simulink model "LQR_2017a"  (R2017a)
settings: Solver=VariableStepAuto  StartTime=0.0  StopTime=4  RelTol=1e-3
values from neighbouring files (symbols this model uses):
  A_obs = A-L*C    [ventilador.m]
  B_obs = [B L]    [ventilador.m]
  C_obs = eye(3)    [ventilador.m]
  D_obs = zeros(3,2)    [ventilador.m]
  K = (tf - t0) / dt    (= 1000)    [pruebaPendulo.m]    (also in ventilador.m = place(A, B, polo_fav))
  Nbar = rscale(sis,K)    [ventilador.m]
undefined symbols (not defined in the file or in its folder): A, B, C, D
settings Model: Creator=jacqu  LastModifiedBy=Gaby
settings SFSimCC: SimUseLocalCustomCode=on
settings RTWCC: RTWUseLocalCustomCode=on

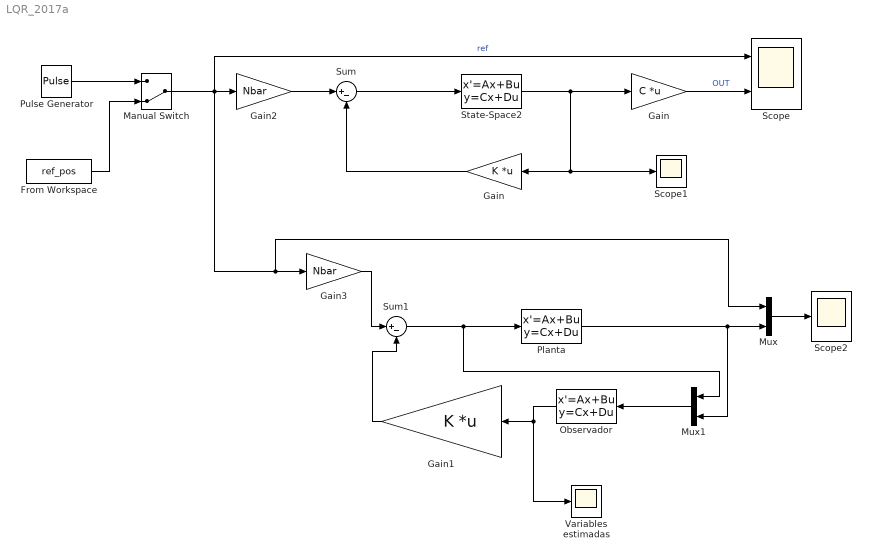
== system LQR_2017a ==
  From Workspace : FromWorkspace  VariableName=ref_pos  OutDataTypeStr=double  SampleTime=0.01
  Gain : Gain  Gain=K  Multiplication=Matrix(K*u) (u vector)
  "Gain " : Gain  Gain=C  Multiplication=Matrix(K*u) (u vector)
  Gain1 : Gain  Gain=K  Multiplication=Matrix(K*u) (u vector)
  Gain2 : Gain  Gain=Nbar
  Gain3 : Gain  Gain=Nbar
  Manual Switch : ManualSwitch  CurrentSetting=0
  Mux : Mux  Inputs=2
  Mux1 : Mux  Inputs=2
  Observador : StateSpace  A=A_obs  B=B_obs  C=C_obs  D=D_obs  X0=0
  Planta : StateSpace  A=A  B=B  C=C  D=D  X0=0
  Pulse Generator : DiscretePulseGenerator  PulseType=Time based  Period=1/0.5  PulseWidth=50
  Scope : Scope  NumInputPorts=2
  Scope1 : Scope
  Scope2 : Scope
  State-Space2 : StateSpace  A=A  B=B  C=eye(3)  D=zeros(3,1)  X0=0
  Sum : Sum  Inputs=|+-
  Sum1 : Sum  Inputs=|+-
  Variables estimadas : Scope
  wires:
  Gain2/1 -> Sum/1
  Sum/1 -> State-Space2/1
  Gain/1 -> Sum/2
  State-Space2/1 -> Scope1/1, Gain/1, "Gain "/1
  "Gain "/1 -> Scope/2  "OUT"
  Pulse Generator/1 -> Manual Switch/1
  From Workspace/1 -> Manual Switch/2
  Manual Switch/1 -> Mux/1, Gain3/1, Scope/1, Gain2/1  "ref"
  Mux/1 -> Scope2/1
  Mux1/1 -> Observador/1
  Observador/1 -> Variables estimadas/1, Gain1/1
  Gain3/1 -> Sum1/1
  Sum1/1 -> Mux1/1, Planta/1
  Gain1/1 -> Sum1/2
  Planta/1 -> Mux1/2, Mux/2
